simulink model "arduino_deploy"  (R2019a)
settings: Solver=FixedStepAuto  StartTime=0.0  StopTime=inf  FixedStep=1/250  RelTol=1e-3  EnableMultiTasking=on
settings Model: ExtModeTrigDuration=2  Creator=marcell  LastModifiedBy=marcellmocher
settings SolverCC: AutoInsertRateTranBlk=on
settings DataIOCC: ReturnWorkspaceOutputs=off
settings OptimizationCC: DefaultUnderspecifiedDataType=single  LifeSpan=1  MaxStackSize=64
settings DebuggingCC: AllowSymbolicDim=off  SFUnexpectedBacktrackingDiag=warning  SFNoUnconditionalDefaultTransitionDiag=warning  SFExecutionAtInitializationDiag=none  ArithmeticOperatorsInVariantConditions=warning
settings HardwareCC: ProdBitPerPointer=32  ProdBitPerSizeT=32  ProdBitPerPtrDiffT=32  ProdLargestAtomicInteger=Long  ProdLargestAtomicFloat=Double  ProdWordSize=32  ProdHWDeviceType=ARM Compatible->ARM Cortex
settings ModelReferenceCC: PropagateSignalLabelsOutOfModel=off
settings SFSimCC: SimUseLocalCustomCode=off  MATLABDynamicMemAlloc=off
settings RTWCC: SystemTargetFile=ert.tlc  HardwareBoard=Arduino Due  TemplateMakefile=ert_default_tmf  RTWUseLocalCustomCode=off  CustomSource=arduino_wrapper.cpp  Toolchain=Arduino ARM  BuildConfiguration=Faster Runs
settings CodeAppCC: IgnoreCustomStorageClasses=off  StateflowObjectComments=on
settings ERTTargetCC: MultiwordLength=2048  SupportContinuousTime=on  SupportNonInlinedSFcns=on  SupportVariableSizeSignals=on  ExtModeStaticAllocSize=24576  ConvertIfToSwitch=off  SuppressUnreachableDefaultCases=off
settings ConfigComp: CovMetricSettings=dw  CovHtmlReporting=on  CovSaveCumulativeToWorkspaceVar=on  CovSaveSingleToWorkspaceVar=on  CovExternalEMLEnable=off

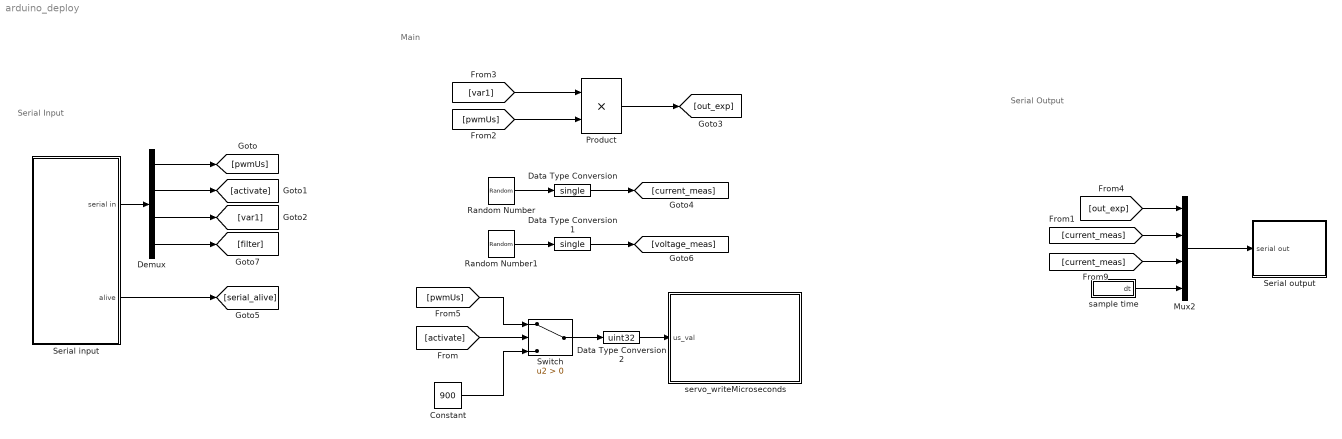
== system arduino_deploy ==
  note: Main
  note: Serial Input
  note: Serial Output
  Constant : Constant  Value=900  OutDataTypeStr=uint32
  Data Type Conversion : DataTypeConversion  OutDataTypeStr=single
  Data Type Conversion1 : DataTypeConversion  OutDataTypeStr=single
  Data Type Conversion2 : DataTypeConversion  OutDataTypeStr=uint32
  Demux : Demux  Outputs=[1 1 1 1]
  Mux2 : Mux  Inputs=[1 1 1 1]
  Product : Product  OutDataTypeStr=single
  Random Number : RandomNumber  SampleTime=1/250
  Random Number1 : RandomNumber  SampleTime=1/250
  Serial input : Subsystem  mask(Serial Input){data_size=4, Baudrate=115200, st_serial=1/250}
      mask prompts: data_size "Data Size"; st_serial "Sample Time"
      mask help: Block for Serial communictaion with gui
  Serial output : Subsystem  mask(Serial output){Baudrate=115200, st_sout=1/125}
      mask prompts: st_sout "Sample Time"
      mask help: Sends values to gui via serial port.
  Switch : Switch  Criteria=u2 > Threshold
  sample time : MATLAB Function  TreatAsAtomicUnit=on
  servo_writeMicroseconds : MATLAB Function  TreatAsAtomicUnit=on  mask{sample_time=1/250, servo_pin=3}
      mask prompts: sample_time "Sample Time"; servo_pin "Pin Number"
  wires:
  Demux/1 -> [pwmUs]
  Demux/2 -> [activate]
  Demux/3 -> [var1]
  Serial input/1(serial in) -> Demux/1
  Mux2/1 -> Serial output/1(serial out)
  [current_meas] -> Mux2/2
  Serial input/2(alive) -> [serial_alive]
  sample time/1(dt) -> Mux2/4
  [current_meas] -> Mux2/3
  Demux/4 -> [filter]
  [pwmUs] -> Product/2
  [var1] -> Product/1
  Product/1 -> [out_exp]
  [out_exp] -> Mux2/1
  Random Number/1 -> Data Type Conversion/1
  Random Number1/1 -> Data Type Conversion1/1
  Data Type Conversion1/1 -> [voltage_meas]
  Data Type Conversion/1 -> [current_meas]
  Data Type Conversion2/1 -> servo_writeMicroseconds/1(us_val)
  Switch/1 -> Data Type Conversion2/1
  Constant/1 -> Switch/3
  [activate] -> Switch/2
  [pwmUs] -> Switch/1

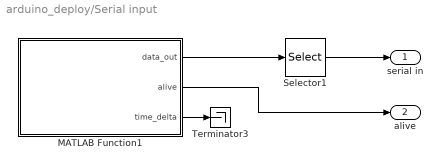
== system arduino_deploy/Serial input ==
  MATLAB Function1 : MATLAB Function  TreatAsAtomicUnit=on
  Selector1 : Selector  InputPortWidth=64  IndexOptions=Index vector (dialog)  Indices=1:data_size  OutputSizes=1
  Terminator3 : Terminator
  serial in : Outport
  alive : Outport  Port=2
  wires:
  MATLAB Function1/1(data_out) -> Selector1/1
  Selector1/1 -> serial in/1
  MATLAB Function1/3(time_delta) -> Terminator3/1
  MATLAB Function1/2(alive) -> alive/1

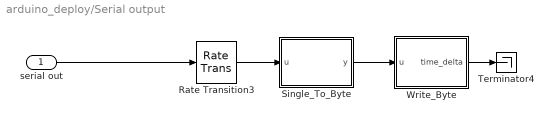
== system arduino_deploy/Serial output ==
  serial out : Inport
  Rate Transition3 : RateTransition  OutPortSampleTime=st_sout
  Single_To_Byte : MATLAB Function  TreatAsAtomicUnit=on
  Terminator4 : Terminator
  Write_Byte : MATLAB Function  TreatAsAtomicUnit=on
  wires:
  Rate Transition3/1 -> Single_To_Byte/1(u)
  Single_To_Byte/1(y) -> Write_Byte/1(u)
  Write_Byte/1(time_delta) -> Terminator4/1
  serial out/1 -> Rate Transition3/1

== matlab function arduino_deploy/servo_writeMicroseconds ==
  settings: updateMethod=DISCRETE  sampleTime=sample_time
  data: us_val input uint32; servo_pin parameter uint8
function servo_writeMicroseconds(us_val, servo_pin)
% /%%
%%%%%%%%%%%%%%%%%%%%%%%%%%%%%%%%%%%%%%%%%%%%%%%%%%%%%%%%%%%%%%%%%%%%%%%%%%%%%%
% @file     servo_writeMicroseconds
% @author   Marcell Mocher
% @version  V0.0.1
% @date     16.6.2016
% @brief    Wrapper for servo wrie microseconds function
%
%
% @requires _get_time
%           _serial_init
%           _serial_available
%           _serial_read
%
%
%%%%%%%%%%%%%%%%%%%%%%%%%%%%%%%%%%%%%%%%%%%%%%%%%%%%%%%%%%%%%%%%%%%%%%%%%%%%%%
% @attention
%
%
%
%
%%%%%%%%%%%%%%%%%%%%%%%%%%%%%%%%%%%%%%%%%%%%%%%%%%%%%%%%%%%%%%%%%%%%%%%%%%%%%%
%/

persistent current_us_val init_flag

if strcmp(coder.target, 'rtw')
    
    if isempty(init_flag)
        init_flag = true;
        current_us_val = uint32(0);
        coder.ceval('_servo_attach',uint8(servo_pin));
    end
    
    
    
    if current_us_val ~= us_val
        coder.ceval('_servo_writeMicroseconds',uint32(us_val));
        current_us_val = us_val;
    end
    
else
    
end

== matlab function arduino_deploy/sample time ==
  data: dt output
function dt = dt()
%#codegen
persistent old_time init_flag

if isempty(init_flag)
    init_flag = true;
    old_time = uint32(0);
end

if strcmp(coder.target, 'rtw')
    T = uint32(0);
    T = coder.ceval('_get_time');
    delta = T - old_time;
    old_time = T;
    dt = single(delta) * 1e-6;
else
    dt = single(1);
end

== matlab function arduino_deploy/Serial input/MATLAB Function1 ==
  settings: updateMethod=DISCRETE  sampleTime=st_serial
  data: data_out output; alive output; time_delta output; Baudrate parameter uint32 size=1
function [data_out,alive,time_delta]  = data_receive(  Baudrate)
% /%%
%%%%%%%%%%%%%%%%%%%%%%%%%%%%%%%%%%%%%%%%%%%%%%%%%%%%%%%%%%%%%%%%%%%%%%%%%%%%%%
% @file     data_receive
% @author   Marcell Mocher
% @version  V0.0.1
% @date     16.6.2016
% @brief    Driver for serial_receive from instrument toolbox
%
%
% @requires _get_time
%           _serial_init
%           _serial_available
%           _serial_read
%
%
%%%%%%%%%%%%%%%%%%%%%%%%%%%%%%%%%%%%%%%%%%%%%%%%%%%%%%%%%%%%%%%%%%%%%%%%%%%%%%
% @attention
%
% 
%
%
%%%%%%%%%%%%%%%%%%%%%%%%%%%%%%%%%%%%%%%%%%%%%%%%%%%%%%%%%%%%%%%%%%%%%%%%%%%%%%
%/



persistent init_flag state head_count idx data length last_update

data_out = single(zeros(64,1));

if strcmp(coder.target, 'rtw')
  
time_start = uint32(0);
time_start = coder.ceval('_get_time');

% Parameter from Mask
baud = uint32(Baudrate); % Standard Baudrate

% Init parameters

if isempty(init_flag)
    init_flag = 0;
    length = uint8(1);
    data = uint8(zeros(512,1));
    idx = uint8(1);
    state = uint8(0);
    head_count = uint8(0);
    last_update = uint32(0);
    coder.ceval('_serial_init',baud);   
end

av = uint8(0);
av = coder.ceval('_serial_available');
if av > 0
    for i = 1:av
        cc = uint8(0);
        cc = coder.ceval('_serial_read');
        switch state
            case 0 %wait for sync 1 (98)
                if cc == 98 
                    state = state + 1;
                    head_count = uint8(1);
                end
            case 1 %wait for sync 2 (98)
                if cc == 98
                    head_count = head_count + 1;
                    if head_count >= 4
                        state = state + 1;
                        idx = uint8(1);
                    end
                else
                    state = uint8(0);
                    head_count = uint8(0);
                end
            case 2 %wait for length
                length = cc;
                state = state + 1;
            case 3 %wait for data
                data(idx) = cc;
                idx = idx + 1;
                if idx > length
                    state = uint8(0);
                    last_update = time_start;
                end
        end % End of switch (state)
        
    end % End for
    
end % End if

data_out(1:length/4) = typecast(data(1:length),'single');

%/* If we have no communication for 1 second*/%
if (time_start - last_update) < 1e6
   alive = true;
else
   alive = false; 
end

time_end = uint32(0);
time_end = coder.ceval('_get_time');
time_delta = time_end - time_start;

else
alive = false;
time_delta = uint32(0);
end
end

== matlab function arduino_deploy/Serial output/Single_To_Byte ==
  settings: updateMethod=DISCRETE  sampleTime=st_sout
  data: u input; y output
function y = SingleToByte(u)
% /%%
%%%%%%%%%%%%%%%%%%%%%%%%%%%%%%%%%%%%%%%%%%%%%%%%%%%%%%%%%%%%%%%%%%%%%%%%%%%%%%
% @file     SingleToByte
% @author   Marcell Mocher
% @version  V0.0.1
% @date     16.6.2016
% @brief    converts single to byte 
%
%%%%%%%%%%%%%%%%%%%%%%%%%%%%%%%%%%%%%%%%%%%%%%%%%%%%%%%%%%%%%%%%%%%%%%%%%%%%%%
% @attention
%
% 
%
%
%%%%%%%%%%%%%%%%%%%%%%%%%%%%%%%%%%%%%%%%%%%%%%%%%%%%%%%%%%%%%%%%%%%%%%%%%%%%%%
%/
u = single(u);
header = uint8(ones(8,1)*97); 
terminator = uint8([13;10]);
len = numel(u);
len_byte = len * 4;
y = uint8(zeros(len_byte+numel(header)+numel(terminator),1));
u_byte = typecast(u,'uint8');
y(1:numel(header)) = header;
for i = 1:numel(u_byte)
   y(i+numel(header)) = u_byte(i) ;
end
y(end-numel(terminator)+1:end) = terminator;

== matlab function arduino_deploy/Serial output/Write_Byte ==
  settings: updateMethod=DISCRETE  sampleTime=st_sout
  data: u input; time_delta output; Baudrate parameter uint32 size=1
function time_delta = write(u, Baudrate)
% /%%
%%%%%%%%%%%%%%%%%%%%%%%%%%%%%%%%%%%%%%%%%%%%%%%%%%%%%%%%%%%%%%%%%%%%%%%%%%%%%%
% @file     
% @author   Marcell Mocher
% @version  V0.0.1
% @date     10.6.2016
% @brief    Example Driver for Serial writing with hardware abstraction layer
%
%%%%%%%%%%%%%%%%%%%%%%%%%%%%%%%%%%%%%%%%%%%%%%%%%%%%%%%%%%%%%%%%%%%%%%%%%%%%%%
% @attention
%
% Requires:  _get_time
%           _serial_init
%           _serial_print
%           _serial_write 
%           _get_time
%
%
%%%%%%%%%%%%%%%%%%%%%%%%%%%%%%%%%%%%%%%%%%%%%%%%%%%%%%%%%%%%%%%%%%%%%%%%%%%%%%
%/
persistent init_flag

if strcmp(coder.target, 'rtw')
    
    time_start = uint32(0);
    time_start = coder.ceval('_get_time');
    
    if isempty(init_flag)
        init_flag = true;
        coder.ceval('_serial_init',uint32(Baudrate));
    end
    len = uint8(numel(u));
    coder.ceval('_serial_write',u,len);
    
    time_end = uint32(0);
    time_end = coder.ceval('_get_time');
    time_delta = time_end - time_start;
else
    time_delta = uint32(0);
end
